simulink model "week2_problem2"  (R2020b)
settings: Solver=VariableStepAuto  StartTime=0.0  StopTime=10.0  RelTol=1e-3
settings Model: Creator=gokul  LastModifiedBy=gokul

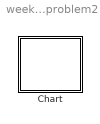
== system week2_problem2 ==
  Chart : Stateflow chart  TreatAsAtomicUnit=on

== stateflow chart week2_problem2/Chart ==
  state Slipping
    entry:
    IeWe=Tin-BeWe-Tcl;
    IvWv=Tcl-WvBv;
    Tcl=sgn(We-Wv)Tfmaxk;
  state Locked
    entry:
    (Ie+Iv)W=Tin-(Be+Bv)W;
    Wv=We=W;
    Tcl=Tf;
  (default) -> Slipping
  Slipping -> Locked
  Locked -> Slipping
